simulink model "EVWITH_BOOSTCONVERTER"  (R2022a)
settings: Solver=ode23t  StartTime=0.0  StopTime=0.025  MaxStep=1e-3  RelTol=1e-3
undefined symbols (not defined in the file): Ion, Lithium
libraries: fl_lib x15, nesl_utility x15, sdl_lib x10, spsSeriesRLCBranchLib x5, spsDiodeLib x4, spsVoltageMeasurementLib x4, ee_lib x4, spsIGBTDiodeLib x4, simulink x3, spsMultimeterLib x3, spsPWMGeneratorDCDCLib x2, spsPowerLib x2
(part 2 of 2)

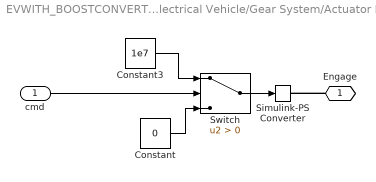
== system EVWITH_BOOSTCONVERTER/Electrical Vehicle/Gear System/Actuator Low ==
  cmd : Inport
  Constant : Constant  Value=0
  Constant3 : Constant  Value=1e7
  Simulink-PS Converter : nesl_utility/Simulink-PS Converter  PhysicalDomain=network_engine_domain  SubClassName=ps_input  LeftPortType=input  RightPortType=output  PseudoPeriodic=off  Frequencies=[]  NoiseDistribution=none  NoiseParameters=[]  Unit=1  AffineConversion=off  FilteringAndDerivatives=provide  SimscapeFilterOrder=1  InputFilterTimeConstant=0.001  UdotUserProvided=0
      settings: SourceProductBaseCode=PW,SS
  Switch : Switch  Criteria=u2 > Threshold  SaturateOnIntegerOverflow=off  InputSameDT=off
  Engage : PMIOPort  Side=Right
  wires:
  Constant/1 -> Switch/3
  cmd/1 -> Switch/2
  Constant3/1 -> Switch/1
  Switch/1 -> Simulink-PS Converter/1
  connections:
  Engage/RConn1 -- Simulink-PS Converter/RConn1

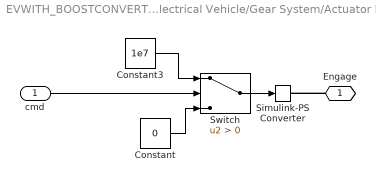
== system EVWITH_BOOSTCONVERTER/Electrical Vehicle/Gear System/Actuator Mid ==
  cmd : Inport
  Constant : Constant  Value=0
  Constant3 : Constant  Value=1e7
  Simulink-PS Converter : nesl_utility/Simulink-PS Converter  PhysicalDomain=network_engine_domain  SubClassName=ps_input  LeftPortType=input  RightPortType=output  PseudoPeriodic=off  Frequencies=[]  NoiseDistribution=none  NoiseParameters=[]  Unit=1  AffineConversion=off  FilteringAndDerivatives=provide  SimscapeFilterOrder=1  InputFilterTimeConstant=0.001  UdotUserProvided=0
      settings: SourceProductBaseCode=PW,SS
  Switch : Switch  Criteria=u2 > Threshold  SaturateOnIntegerOverflow=off  InputSameDT=off
  Engage : PMIOPort  Side=Right
  wires:
  Switch/1 -> Simulink-PS Converter/1
  Constant3/1 -> Switch/1
  cmd/1 -> Switch/2
  Constant/1 -> Switch/3
  connections:
  Engage/RConn1 -- Simulink-PS Converter/RConn1
